simulink model "Code_of_Section_IV_A"  (R2020a)
settings: Solver=FixedStepAuto  StartTime=0.0  StopTime=2  RelTol=1e-5  EnableMultiTasking=on
settings Model: Creator=13018  LastModifiedBy=Administrator
settings DataIOCC: ReturnWorkspaceOutputs=off
settings OptimizationCC: LifeSpan=inf
settings DebuggingCC: SFUnexpectedBacktrackingDiag=warning  SFNoUnconditionalDefaultTransitionDiag=warning  ArithmeticOperatorsInVariantConditions=warning
settings SFSimCC: SimUseLocalCustomCode=off  CustomCodeUndefinedFunction=UseInterfaceOnly
settings RTWCC: RTWUseLocalCustomCode=off
settings CodeAppCC: StateflowObjectComments=on
settings GRTTargetCC: TargetLangStandard=C89/C90 (ANSI)
settings ConfigComp: CovMetricSettings=dw  CovHtmlReporting=on  CovSaveCumulativeToWorkspaceVar=on  CovSaveSingleToWorkspaceVar=on  CovExternalEMLEnable=off

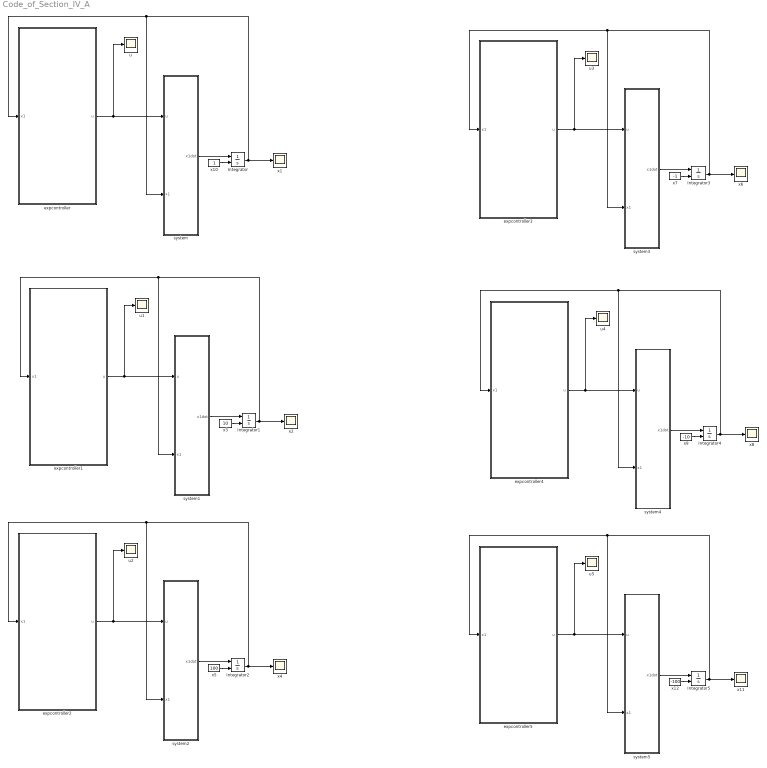
== system Code_of_Section_IV_A ==
  Integrator{,1..5} (6 alike) : Integrator  InitialConditionSource=external
  expcontroller : MATLAB Function  TreatAsAtomicUnit=on
  expcontroller1 : MATLAB Function  TreatAsAtomicUnit=on
  expcontroller2 : MATLAB Function  TreatAsAtomicUnit=on
  expcontroller3 : MATLAB Function  TreatAsAtomicUnit=on
  expcontroller4 : MATLAB Function  TreatAsAtomicUnit=on
  expcontroller5 : MATLAB Function  TreatAsAtomicUnit=on
  system : MATLAB Function  TreatAsAtomicUnit=on
  system1 : MATLAB Function  TreatAsAtomicUnit=on
  system2 : MATLAB Function  TreatAsAtomicUnit=on
  system3 : MATLAB Function  TreatAsAtomicUnit=on
  system4 : MATLAB Function  TreatAsAtomicUnit=on
  system5 : MATLAB Function  TreatAsAtomicUnit=on
  u{,1..5} (6 alike) : Scope
  x{1..2,4,6,8,11} (6 alike) : Scope
  x10 : Constant  VectorParams1D=off  SampleTime=-1
  x12 : Constant  Value=-100  VectorParams1D=off  SampleTime=-1
  x3 : Constant  Value=10  VectorParams1D=off  SampleTime=-1
  x5 : Constant  Value=100  VectorParams1D=off  SampleTime=-1
  x7 : Constant  Value=-1  VectorParams1D=off  SampleTime=-1
  x9 : Constant  Value=-10  VectorParams1D=off  SampleTime=-1
  wires:
  system/1(x1dot) -> Integrator/1
  x10/1 -> Integrator/2
  Integrator/1 -> system/2(x1), expcontroller/1(x1), x1/1
  expcontroller/1(u) -> u/1, system/1(u)
  x3/1 -> Integrator1/2
  system1/1(x1dot) -> Integrator1/1
  expcontroller1/1(u) -> u1/1, system1/1(u)
  Integrator1/1 -> system1/2(x1), expcontroller1/1(x1), x2/1
  x5/1 -> Integrator2/2
  system2/1(x1dot) -> Integrator2/1
  expcontroller2/1(u) -> u2/1, system2/1(u)
  Integrator2/1 -> system2/2(x1), expcontroller2/1(x1), x4/1
  x12/1 -> Integrator5/2
  Integrator4/1 -> system4/2(x1), expcontroller4/1(x1), x8/1
  system4/1(x1dot) -> Integrator4/1
  expcontroller4/1(u) -> u4/1, system4/1(u)
  Integrator3/1 -> system3/2(x1), expcontroller3/1(x1), x6/1
  x7/1 -> Integrator3/2
  x9/1 -> Integrator4/2
  system5/1(x1dot) -> Integrator5/1
  Integrator5/1 -> system5/2(x1), expcontroller5/1(x1), x11/1
  system3/1(x1dot) -> Integrator3/1
  expcontroller5/1(u) -> u5/1, system5/1(u)
  expcontroller3/1(u) -> u3/1, system3/1(u)

== matlab function Code_of_Section_IV_A/system1 ==
  data: u input; x1 input; x1dot output
function x1dot  = fcn(u,x1)
x1dot=x1+u;
end

== matlab function Code_of_Section_IV_A/expcontroller2 ==
  data: u output; x1 input
function u   = fcn(x1)
Tc=1;
x1s=0.1;
x1c=100;

u=-log(x1c/x1s)/(Tc)*x1-x1;

end

== matlab function Code_of_Section_IV_A/system2 ==
  data: u input; x1 input; x1dot output
function x1dot  = fcn(u,x1)
x1dot=x1+u;
end

== matlab function Code_of_Section_IV_A/expcontroller3 ==
  data: u output; x1 input
function u   = fcn(x1)
Tc=1;
x1s=0.1;
x1c=100;

u=-log(x1c/x1s)/(Tc)*x1-x1;

end

== matlab function Code_of_Section_IV_A/expcontroller4 ==
  data: u output; x1 input
function u   = fcn(x1)
Tc=1;
x1s=0.1;
x1c=100;

u=-log(x1c/x1s)/(Tc)*x1-x1;

end

== matlab function Code_of_Section_IV_A/expcontroller5 ==
  data: u output; x1 input
function u   = fcn(x1)
Tc=1;
x1s=0.1;
x1c=100;

u=-log(x1c/x1s)/(Tc)*x1-x1;

end

== matlab function Code_of_Section_IV_A/system3 ==
  data: u input; x1 input; x1dot output
function x1dot  = fcn(u,x1)
x1dot=x1+u;
end

== matlab function Code_of_Section_IV_A/system4 ==
  data: u input; x1 input; x1dot output
function x1dot  = fcn(u,x1)
x1dot=x1+u;
end

== matlab function Code_of_Section_IV_A/system5 ==
  data: u input; x1 input; x1dot output
function x1dot  = fcn(u,x1)
x1dot=x1+u;
end

== matlab function Code_of_Section_IV_A/expcontroller1 ==
  data: u output; x1 input
function u   = fcn(x1)
Tc=1;
x1s=0.1;
x1c=100;

u=-log(x1c/x1s)/(Tc)*x1-x1;

end

== matlab function Code_of_Section_IV_A/system ==
  data: u input; x1 input; x1dot output
function x1dot  = fcn(u,x1)
x1dot=x1+u;
end

== matlab function Code_of_Section_IV_A/expcontroller ==
  data: u output; x1 input
function u   = fcn(x1)
Tc=1;
x1s=0.1;
x1c=100;

u=-log(x1c/x1s)/(Tc)*x1-x1;

end
